simulink model "RT_dennis"  (R2013a)
settings: Solver=ode45  StartTime=0.0  StopTime=10.0  RelTol=1e-3
settings Model: Creator=mainster  LastModifiedBy=mainster
settings DebuggingCC: SolverPrmCheckMsg=none

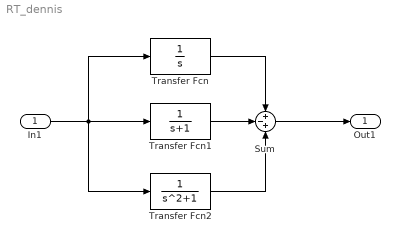
== system RT_dennis ==
  In1 : Inport
  Sum : Sum  Inputs=+-+
  Transfer Fcn : TransferFcn  Denominator=[1 0]
  Transfer Fcn1 : TransferFcn  Denominator=[1 1]
  Transfer Fcn2 : TransferFcn  Denominator=[1 0 1]
  Out1 : Outport
  wires:
  Transfer Fcn/1 -> Sum/1
  Transfer Fcn1/1 -> Sum/2
  Transfer Fcn2/1 -> Sum/3
  In1/1 -> Transfer Fcn2/1, Transfer Fcn/1, Transfer Fcn1/1
  Sum/1 -> Out1/1
